simulink model "Ex6_4"  (Simulink 6.0)
settings: Solver=FixedStepDiscrete  SolverMode=SingleTasking  StartTime=0.0  StopTime=Ts*100  FixedStep=Ts  RelTol=1e-3  AbsTol=1e-6
values from neighbouring files (symbols this model uses):
  Ampl = 10^(Amp_dB/20)-pi/1024    (= 0.704877822808)    [Ex6_6Launch.m]
  Feedforward = 1    [Ex6_6Launch.m]
  finrad = Fin*2*pi    (= 201322.092971)    [Ex6_6Launch.m]
  Ncomp = 7    [Ex6_6Launch.m]
  Ts = 1/Fs    (= 3.54308390023e-07)    [Ex6_6Launch.m]
  VrefN = -1    [Ex6_6Launch.m]
  VrefP = 1    [Ex6_6Launch.m]
undefined symbols (not defined in the file or in its folder): Quantiz
settings Model: Creator=francomaloberti  LastModifiedBy=Cri  ExtModeAutoUpdateStatusClock=off
settings DataIOCC: LimitDataPoints=off  SignalLoggingName=sigsOut
settings OptimizationCC: BooleanDataType=off  InlineInvariantSignals=off
settings DebuggingCC: SolverPrmCheckMsg=none
settings HardwareCC: TargetUnknown=on

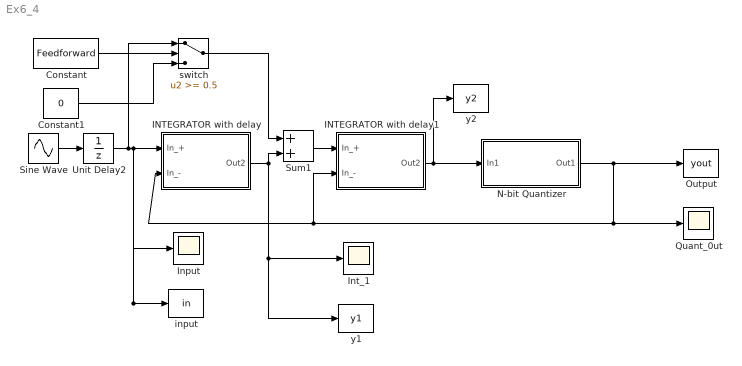
== system Ex6_4 ==
  Constant : Constant  Value=Feedforward
  Constant1 : Constant  Value=0
  INTEGRATOR with delay : Subsystem
      mask Display:
      | patch([10 40 10 10], [0 20 40 0],[1 0 1])
      | plot([10 40 10 10], [0 20 40 0])
      | plot([0 10], [8 8])
      | plot([0 10], [28 28])
      | dpoly([0 1], [1 -1], 'z-')
      | port_label('input', 1, '+')
      | port_label('input', 2, '-')
  INTEGRATOR with delay1 : Subsystem
      mask Display:
      | patch([10 40 10 10], [0 20 40 0],[1 0 1])
      | plot([10 40 10 10], [0 20 40 0])
      | plot([0 10], [8 8])
      | plot([0 10], [28 28])
      | dpoly([0 1], [1 -1], 'z-')
      | port_label('input', 1, '+')
      | port_label('input', 2, '-')
  Input : Scope
      settings: TimeRange=0.003  YMin=-0.4  YMax=0.4
  Int_1 : Scope
      settings: TimeRange=0.003  YMin=-0.4  YMax=0.4  SaveName=ScopeData3
  N-bit Quantizer : Subsystem
      mask Display: color('green'),disp('N-bit QUANTIZER');
  Output : ToWorkspace  VariableName=yout  SampleTime=Ts  SaveFormat=Array
  Quant_0ut : Scope
  Sine Wave : Sin  Amplitude=Ampl  Frequency=finrad
  Sum1 : Sum  SaturateOnIntegerOverflow=on  InputSameDT=on
  Unit Delay2 : UnitDelay  SampleTime=Ts
  input : ToWorkspace  VariableName=in  SampleTime=Ts  SaveFormat=Array
  switch : Switch  Threshold=0.5
  y1 : ToWorkspace  VariableName=y1  SampleTime=Ts  SaveFormat=Array
  y2 : ToWorkspace  VariableName=y2  SampleTime=Ts  SaveFormat=Array
  wires:
  Sine Wave/1 -> Unit Delay2/1
  Unit Delay2/1 -> Input/1, input/1, INTEGRATOR with delay/1(In_+), switch/1
  INTEGRATOR with delay1/1(Out2) -> y2/1, N-bit Quantizer/1(In1)
  INTEGRATOR with delay/1(Out2) -> Sum1/2, Int_1/1, y1/1
  Sum1/1 -> INTEGRATOR with delay1/1(In_+)
  switch/1 -> Sum1/1
  Constant/1 -> switch/2
  Constant1/1 -> switch/3
  N-bit Quantizer/1(Out1) -> Output/1, Quant_0ut/1, INTEGRATOR with delay1/2(In_-), INTEGRATOR with delay/2(In_-)

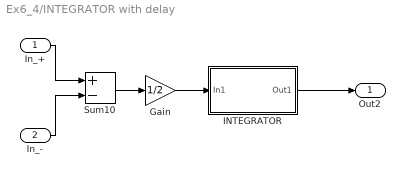
== system Ex6_4/INTEGRATOR with delay ==
  In_+ : Inport  Port=1  LatchInput=off
  In_- : Inport  Port=2  LatchInput=off
  Gain : Gain  Gain=1/2  SaturateOnIntegerOverflow=on
  INTEGRATOR : Subsystem
      mask Display:
      | patch([0 20 0 0], [0 10 20 0],[0 1 0])
      | text(5,10,'\bf\int','texmode','on')
      | plot([0 20 0 0], [0 10 20 0])
  Sum10 : Sum  Inputs=+-  SaturateOnIntegerOverflow=on  InputSameDT=on
  Out2 : Outport
  wires:
  Sum10/1 -> Gain/1
  In_-/1 -> Sum10/2
  In_+/1 -> Sum10/1
  Gain/1 -> INTEGRATOR/1(In1)
  INTEGRATOR/1(Out1) -> Out2/1

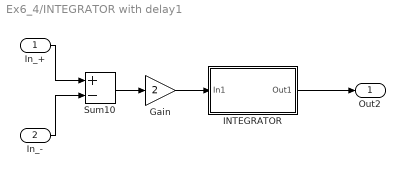
== system Ex6_4/INTEGRATOR with delay1 ==
  In_+ : Inport  Port=1  LatchInput=off
  In_- : Inport  Port=2  LatchInput=off
  Gain : Gain  Gain=2  SaturateOnIntegerOverflow=on
  INTEGRATOR : Subsystem
      mask Display:
      | patch([0 20 0 0], [0 10 20 0],[0 1 0])
      | text(5,10,'\bf\int','texmode','on')
      | plot([0 20 0 0], [0 10 20 0])
  Sum10 : Sum  Inputs=+-  SaturateOnIntegerOverflow=on  InputSameDT=on
  Out2 : Outport
  wires:
  Sum10/1 -> Gain/1
  In_-/1 -> Sum10/2
  In_+/1 -> Sum10/1
  Gain/1 -> INTEGRATOR/1(In1)
  INTEGRATOR/1(Out1) -> Out2/1

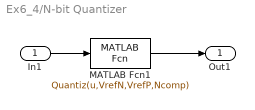
== system Ex6_4/N-bit Quantizer ==
  In1 : Inport  Port=1  LatchInput=off
  MATLAB Fcn1 : MATLABFcn  MATLABFcn=Quantiz(u,VrefN,VrefP,Ncomp)  OutputDimensions=1  Output1D=off  SampleTime=Ts
  Out1 : Outport
  wires:
  In1/1 -> MATLAB Fcn1/1
  MATLAB Fcn1/1 -> Out1/1

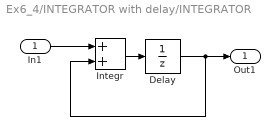
== system Ex6_4/INTEGRATOR with delay/INTEGRATOR ==
  In1 : Inport  Port=1  LatchInput=off
  Delay : UnitDelay  SampleTime=Ts
  Integr : Sum  OutScaling=2^-10
  Out1 : Outport
  wires:
  In1/1 -> Integr/1
  Integr/1 -> Delay/1
  Delay/1 -> Out1/1, Integr/2

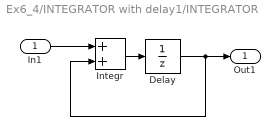
== system Ex6_4/INTEGRATOR with delay1/INTEGRATOR ==
  In1 : Inport  Port=1  LatchInput=off
  Delay : UnitDelay  SampleTime=Ts
  Integr : Sum  OutScaling=2^-10
  Out1 : Outport
  wires:
  In1/1 -> Integr/1
  Integr/1 -> Delay/1
  Delay/1 -> Out1/1, Integr/2
